simulink model "flow_t"  (Simulink 6.0)
settings: Solver=ode45  SolverMode=SingleTasking  StartTime=0.0  StopTime=10.0  RelTol=1e-3  AbsTol=1e-6
undefined symbols (not defined in the file or in its folder): STime
settings Model: Creator=Administrator  LastModifiedBy=Administrator  ExtModeTrigMode=oneshot  ExtModeArmWhenConnect=off
settings DataIOCC: LimitDataPoints=off
settings OptimizationCC: BlockReduction=off  BooleanDataType=off  InlineInvariantSignals=off  ExpressionDepthLimit=2147483647  SimCompilerOptimization=Off
settings DebuggingCC: SaveWithParameterizedLinksMsg=none  SolverPrmCheckMsg=none  MultiTaskDSMMsg=warning  MultiTaskCondExecSysMsg=none  FcnCallInpInsideContextMsg=Use local settings  StateNameClashWarn=warning  StrictBusMsg=None
settings HardwareCC: TargetHWDeviceType=32-bit Generic  TargetUnknown=on  ProdEqTarget=off
settings RTWCC: IncludeERTFirstTime=on  RTWCompilerOptimization=Off
settings CodeAppCC: CustomSymbolStrType=$N$R$M

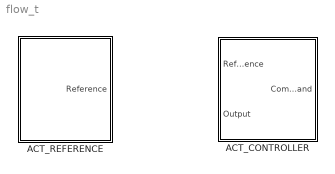
== system flow_t ==
  ACT_CONTROLLER : Subsystem
  ACT_REFERENCE : Subsystem

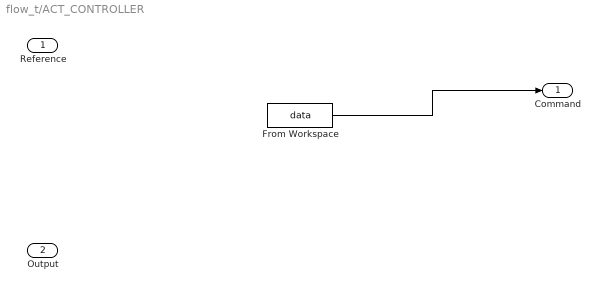
== system flow_t/ACT_CONTROLLER ==
  Reference : Inport
  Output : Inport  Port=2
  From Workspace : FromWorkspace  VariableName=data  SampleTime=0
  Command : Outport
  wires:
  From Workspace/1 -> Command/1

== system flow_t/ACT_REFERENCE ==
  note: If you want to change the reference signals open the left subsystem.
      | Some references are already inserted. You can remove them or,
      | if you like,  insert new reference functions by copy and paste objects
      | from the top-right block. You can also modify such objects or write new ones.
  First Input : Subsystem
  Other References : Subsystem
  Reference : Outport  InitialOutput=0
  wires:
  First Input/1(Out1) -> Reference/1

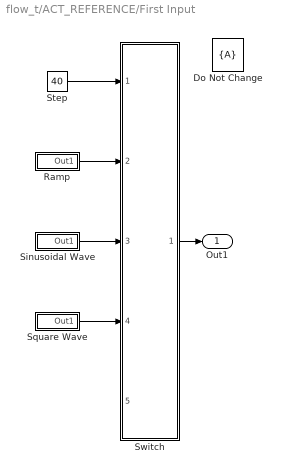
== system flow_t/ACT_REFERENCE/First Input ==
  Do Not Change : GotoTagVisibility
  Ramp : Subsystem
  Sinusoidal Wave : Subsystem
  Square Wave : Subsystem
  Step : Constant  Value=40
  Switch : Subsystem
  Out1 : Outport  InitialOutput=0
  wires:
  Step/1 -> Switch/1(Ref 1)
  Ramp/1(Out1) -> Switch/2(Ref 2)
  Sinusoidal Wave/1(Out1) -> Switch/3(Ref 3)
  Switch/1(Out1) -> Out1/1
  Square Wave/1(Out1) -> Switch/4(Ref 4)

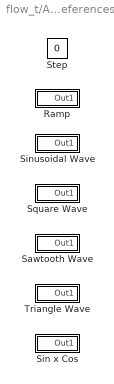
== system flow_t/ACT_REFERENCE/Other References ==
  Ramp : Subsystem
  Sawtooth Wave : Subsystem
  Sin x Cos : Subsystem
  Sinusoidal Wave : Subsystem
  Square Wave : Subsystem
  Step : Constant  Value=0
  Triangle Wave : Subsystem

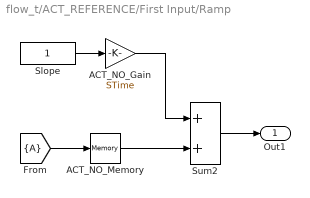
== system flow_t/ACT_REFERENCE/First Input/Ramp ==
  ACT_NO_Gain : Gain  Gain=STime  SaturateOnIntegerOverflow=on
  ACT_NO_Memory : Memory  InheritSampleTime=on
  Slope : Constant
  Sum2 : Sum  SaturateOnIntegerOverflow=on  InputSameDT=on
  Out1 : Outport  InitialOutput=0
  wires:
  ACT_NO_Gain/1 -> Sum2/1
  Slope/1 -> ACT_NO_Gain/1
  [A] -> ACT_NO_Memory/1
  ACT_NO_Memory/1 -> Sum2/2
  Sum2/1 -> Out1/1

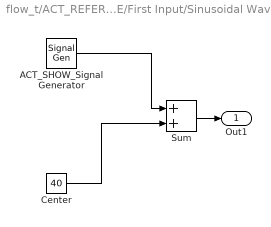
== system flow_t/ACT_REFERENCE/First Input/Sinusoidal Wave ==
  ACT_SHOW_Signal Generator : SignalGenerator  Amplitude=10  Frequency=0.1
  Center : Constant  Value=40
  Sum : Sum  SaturateOnIntegerOverflow=on  InputSameDT=on
  Out1 : Outport  InitialOutput=0
  wires:
  Sum/1 -> Out1/1
  Center/1 -> Sum/2
  ACT_SHOW_Signal Generator/1 -> Sum/1

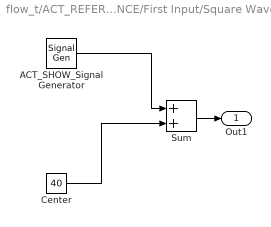
== system flow_t/ACT_REFERENCE/First Input/Square Wave ==
  ACT_SHOW_Signal Generator : SignalGenerator  WaveForm=square  Amplitude=10  Frequency=0.1
  Center : Constant  Value=40
  Sum : Sum  SaturateOnIntegerOverflow=on  InputSameDT=on
  Out1 : Outport  InitialOutput=0
  wires:
  Sum/1 -> Out1/1
  Center/1 -> Sum/2
  ACT_SHOW_Signal Generator/1 -> Sum/1

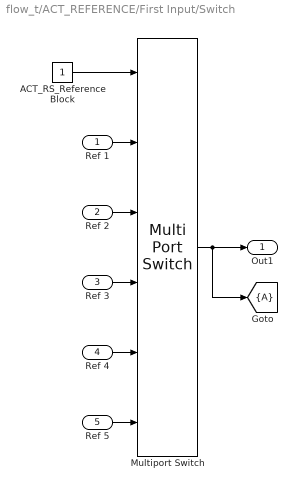
== system flow_t/ACT_REFERENCE/First Input/Switch ==
  Ref 1 : Inport
  Ref 2 : Inport  Port=2
  Ref 3 : Inport  Port=3
  Ref 4 : Inport  Port=4
  Ref 5 : Inport  Port=5
  ACT_RS_Reference Block : Constant
  Multiport Switch : MultiPortSwitch  Inputs=5  SaturateOnIntegerOverflow=on  InputSameDT=on
  Out1 : Outport  InitialOutput=0
  tag scope: A=scoped
  wires:
  Ref 5/1 -> Multiport Switch/6
  Ref 4/1 -> Multiport Switch/5
  Ref 3/1 -> Multiport Switch/4
  Ref 2/1 -> Multiport Switch/3
  Ref 1/1 -> Multiport Switch/2
  ACT_RS_Reference Block/1 -> Multiport Switch/1
  Multiport Switch/1 -> Out1/1, [A]

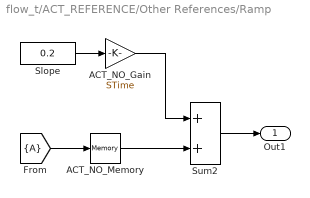
== system flow_t/ACT_REFERENCE/Other References/Ramp ==
  ACT_NO_Gain : Gain  Gain=STime  SaturateOnIntegerOverflow=on
  ACT_NO_Memory : Memory  InheritSampleTime=on
  Slope : Constant  Value=0.2
  Sum2 : Sum  SaturateOnIntegerOverflow=on  InputSameDT=on
  Out1 : Outport  InitialOutput=0
  wires:
  Sum2/1 -> Out1/1
  ACT_NO_Memory/1 -> Sum2/2
  [A] -> ACT_NO_Memory/1
  Slope/1 -> ACT_NO_Gain/1
  ACT_NO_Gain/1 -> Sum2/1

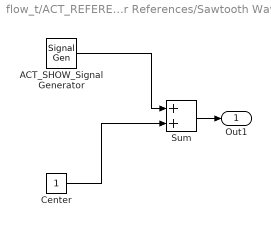
== system flow_t/ACT_REFERENCE/Other References/Sawtooth Wave ==
  ACT_SHOW_Signal Generator : SignalGenerator  WaveForm=sawtooth  Amplitude=0.3  Frequency=0.01
  Center : Constant
  Sum : Sum  SaturateOnIntegerOverflow=on  InputSameDT=on
  Out1 : Outport  InitialOutput=0
  wires:
  Sum/1 -> Out1/1
  Center/1 -> Sum/2
  ACT_SHOW_Signal Generator/1 -> Sum/1

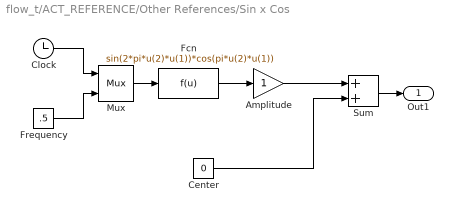
== system flow_t/ACT_REFERENCE/Other References/Sin x Cos ==
  Amplitude : Gain  SaturateOnIntegerOverflow=on
  Center : Constant  Value=0
  Clock : Clock
      settings: Decimation=10
  Fcn : Fcn  Expr=sin(2*pi*u(2)*u(1))*cos(pi*u(2)*u(1))
  Frequency : Constant  Value=.5
  Mux : Mux  Inputs=2
  Sum : Sum  SaturateOnIntegerOverflow=on  InputSameDT=on
  Out1 : Outport  InitialOutput=0
  wires:
  Mux/1 -> Fcn/1
  Clock/1 -> Mux/1
  Frequency/1 -> Mux/2
  Fcn/1 -> Amplitude/1
  Amplitude/1 -> Sum/1
  Sum/1 -> Out1/1
  Center/1 -> Sum/2

== system flow_t/ACT_REFERENCE/Other References/Sinusoidal Wave ==
  ACT_SHOW_Signal Generator : SignalGenerator
  Center : Constant  Value=0
  Sum : Sum  SaturateOnIntegerOverflow=on  InputSameDT=on
  Out1 : Outport  InitialOutput=0
  wires:
  Sum/1 -> Out1/1
  Center/1 -> Sum/2
  ACT_SHOW_Signal Generator/1 -> Sum/1

== system flow_t/ACT_REFERENCE/Other References/Square Wave ==
  ACT_SHOW_Signal Generator : SignalGenerator  WaveForm=square
  Center : Constant  Value=0
  Sum : Sum  SaturateOnIntegerOverflow=on  InputSameDT=on
  Out1 : Outport  InitialOutput=0
  wires:
  ACT_SHOW_Signal Generator/1 -> Sum/1
  Center/1 -> Sum/2
  Sum/1 -> Out1/1

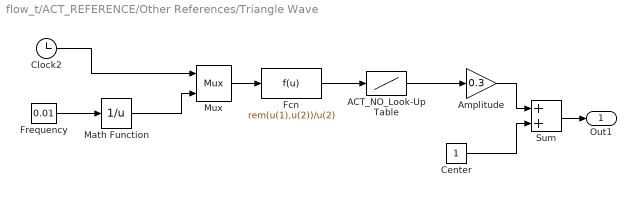
== system flow_t/ACT_REFERENCE/Other References/Triangle Wave ==
  ACT_NO_Look-Up Table : Lookup  InputValues=[0 0.5 1]  OutputValues=[-1 1 -1]  SaturateOnIntegerOverflow=on
  Amplitude : Gain  Gain=0.3  SaturateOnIntegerOverflow=on
  Center : Constant
  Clock2 : Clock
      settings: Decimation=10
  Fcn : Fcn  Expr=rem(u(1),u(2))/u(2)
  Frequency : Constant  Value=0.01
  Math Function : Math  Operator=reciprocal  SaturateOnIntegerOverflow=on
  Mux : Mux  Inputs=2
  Sum : Sum  SaturateOnIntegerOverflow=on  InputSameDT=on
  Out1 : Outport  InitialOutput=0
  wires:
  Clock2/1 -> Mux/1
  Sum/1 -> Out1/1
  Center/1 -> Sum/2
  Amplitude/1 -> Sum/1
  ACT_NO_Look-Up Table/1 -> Amplitude/1
  Fcn/1 -> ACT_NO_Look-Up Table/1
  Mux/1 -> Fcn/1
  Frequency/1 -> Math Function/1
  Math Function/1 -> Mux/2
